simulink model "Portefolio_2_2"  (Simulink 7.5)
settings: Solver=ode45  StartTime=0.0  StopTime=20  MaxStep=0.01  RelTol=1e-3
values from neighbouring files (symbols this model uses):
  A = 1/(k1^2 - k4^2)*[k3*k4 k1*k3; k1*k3 k3*k4]    [portfolie_2_better.m]
  b = 0.26    [portfolie_2_better.m]    (also in portfolie_2_lol.m)
  B = 1/(k1^2 - k4^2)*[(-k2)*k4 (-k1)*k2; (-k1)*k2 (-k2)*k4]    [portfolie_2_better.m]
  C = [1 0; 0 1]    [portfolie_2_better.m]
  K = [35 10; 10 35]    [portfolie_2_better.m]
  L = 4 * K    [portfolie_2_better.m]
  r = 0.1    [portfolie_2_better.m]    (also in portfolie_2_lol.m)
  sys = ss(A,B,C,D)    [portfolie_2_better.m]    (also in portfolie_2_lol.m = canon(G,'modal'))
libraries: simulink x3
settings Model: Creator=Jeppe Pedersen  LastModifiedBy=Jeppe Pedersen

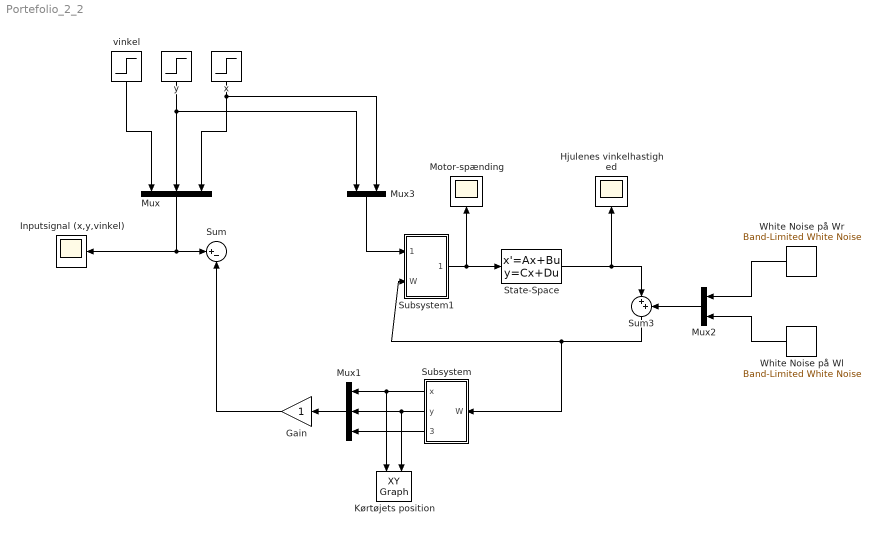
== system Portefolio_2_2 ==
  Gain : Gain  ParameterDataType=fixdt(1, 16)  ParameterScaling=2^0  OutDataType=fixdt(1, 16)  OutScaling=2^0
  Hjulenes vinkelhastighed : Scope
  Inputsignal (x,y,vinkel) : Scope
  Kørtøjets position : simulink/Sinks/XY Graph  SystemSampleTime=-1  xmin=-10  xmax=10  ymin=-10  ymax=10  st=-1
  Motor-spænding : Scope
      settings: SaveName=ScopeData2
  Mux : Mux  Inputs=3
  Mux1 : Mux  Inputs=3
  Mux2 : Mux  Inputs=2
  Mux3 : Mux  Inputs=2
  State-Space : StateSpace  A=sys.A  B=sys.B  C=sys.C  D=sys.D
  Subsystem : Subsystem
  Subsystem1 : Subsystem
  Sum : Sum  Inputs=|+-  OutDataType=fixdt(1, 16)  OutScaling=2^0
  Sum3 : Sum  Inputs=|++  OutDataType=fixdt(1, 16)  OutScaling=2^0
  White Noise på Wl : simulink/Sources/Band-Limited White Noise  SystemSampleTime=-1  Cov=0  Ts=0.01  seed=[27741]
  White Noise på Wr : simulink/Sources/Band-Limited White Noise  SystemSampleTime=-1  Cov=0  Ts=0.01  seed=[23341]
  vinkel : Step  After=5  SampleTime=0
  x : Step  After=5  SampleTime=0
  y : Step  After=4  SampleTime=0
  wires:
  State-Space/1 -> Hjulenes vinkelhastighed/1, Sum3/1
  Mux/1 -> Inputsignal (x,y,vinkel)/1, Sum/1
  Sum3/1 -> Subsystem/1(W), Subsystem1/2(W)
  Subsystem1/1(u [V]) -> State-Space/1, Motor-spænding/1
  Mux1/1 -> Gain/1
  Subsystem/1(x) -> Mux1/1, Kørtøjets position/1
  Subsystem/2(y) -> Mux1/2, Kørtøjets position/2
  Subsystem/3(vinkel) -> Mux1/3
  Gain/1 -> Sum/2
  x/1 -> Mux/3, Mux3/2
  y/1 -> Mux/2, Mux3/1
  vinkel/1 -> Mux/1
  White Noise på Wr/1 -> Mux2/1
  White Noise på Wl/1 -> Mux2/2
  Mux2/1 -> Sum3/2
  Mux3/1 -> Subsystem1/1(Wd)

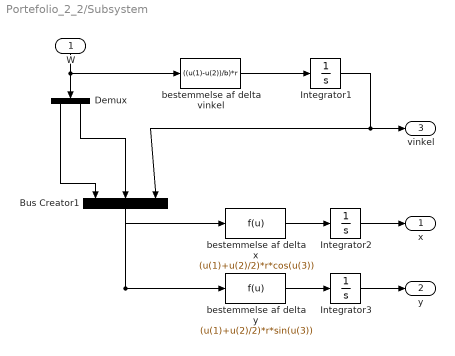
== system Portefolio_2_2/Subsystem ==
  W : Inport
  Bus Creator1 : BusCreator  Inputs=3
  Demux : Demux  Outputs=2
  Integrator1 : Integrator
  Integrator2 : Integrator
  Integrator3 : Integrator
  bestemmelse af delta vinkel : Fcn  Expr=((u(1)-u(2))/b)*r
  bestemmelse af delta x : Fcn  Expr=(u(1)+u(2)/2)*r*cos(u(3))
  bestemmelse af delta y : Fcn  Expr=(u(1)+u(2)/2)*r*sin(u(3))
  x : Outport
  y : Outport  Port=2
  vinkel : Outport  Port=3
  wires:
  Demux/1 -> Bus Creator1/1
  Demux/2 -> Bus Creator1/2
  Bus Creator1/1 -> bestemmelse af delta x/1, bestemmelse af delta y/1
  Integrator3/1 -> y/1
  bestemmelse af delta y/1 -> Integrator3/1
  Integrator2/1 -> x/1
  bestemmelse af delta x/1 -> Integrator2/1
  Integrator1/1 -> Bus Creator1/3, vinkel/1
  bestemmelse af delta vinkel/1 -> Integrator1/1
  W/1 -> Demux/1, bestemmelse af delta vinkel/1

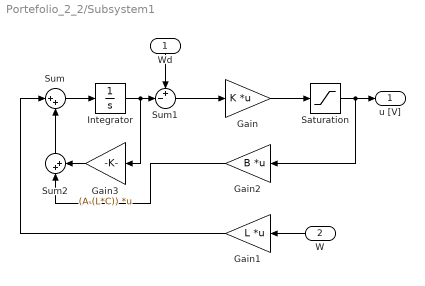
== system Portefolio_2_2/Subsystem1 ==
  Wd : Inport
  W : Inport  Port=2
  Gain : Gain  Gain=K  Multiplication=Matrix(K*u)  ParameterDataType=fixdt(1, 16)  ParameterScaling=2^0  OutDataType=fixdt(1, 16)  OutScaling=2^0
  Gain1 : Gain  Gain=L  Multiplication=Matrix(K*u)  ParameterDataType=fixdt(1, 16)  ParameterScaling=2^0  OutDataType=fixdt(1, 16)  OutScaling=2^0
  Gain2 : Gain  Gain=B  Multiplication=Matrix(K*u)  ParameterDataType=fixdt(1, 16)  ParameterScaling=2^0  OutDataType=fixdt(1, 16)  OutScaling=2^0
  Gain3 : Gain  Gain=(A-(L*C))  Multiplication=Matrix(K*u)  ParameterDataType=fixdt(1, 16)  ParameterScaling=2^0  OutDataType=fixdt(1, 16)  OutScaling=2^0
  Integrator : Integrator
  Saturation : Saturate  UpperLimit=12  LowerLimit=-12  OutDataType=fixdt(1, 16)  OutScaling=2^0
  Sum : Sum  Inputs=|++  OutDataType=fixdt(1, 16)  OutScaling=2^0
  Sum1 : Sum  Inputs=+-|  OutDataType=fixdt(1, 16)  OutScaling=2^0  InputSameDT=on
  Sum2 : Sum  Inputs=|++  OutDataType=fixdt(1, 16)  OutScaling=2^0
  u [V] : Outport
  wires:
  Gain/1 -> Saturation/1
  Gain1/1 -> Sum/1
  Sum/1 -> Integrator/1
  Integrator/1 -> Sum1/2, Gain3/1
  Sum1/1 -> Gain/1
  Gain3/1 -> Sum2/2
  Gain2/1 -> Sum2/1
  Sum2/1 -> Sum/2
  Saturation/1 -> Gain2/1, u [V]/1
  Wd/1 -> Sum1/1
  W/1 -> Gain1/1
